simulink subsystem "HousegenTransform"  (R2023b)
settings: Solver=VariableStepAuto  StartTime=0.0  StopTime=10.0  RelTol=1e-3
libraries: hdlsllib x1
settings Model: Creator=Koche  LastModifiedBy=Koche

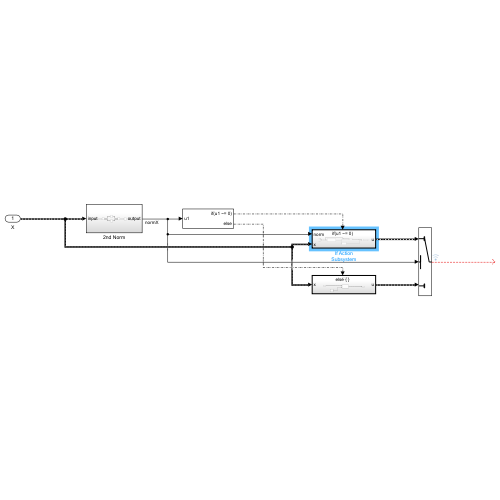
[thumbnail: Simulink's stored preview of the top-level diagram]
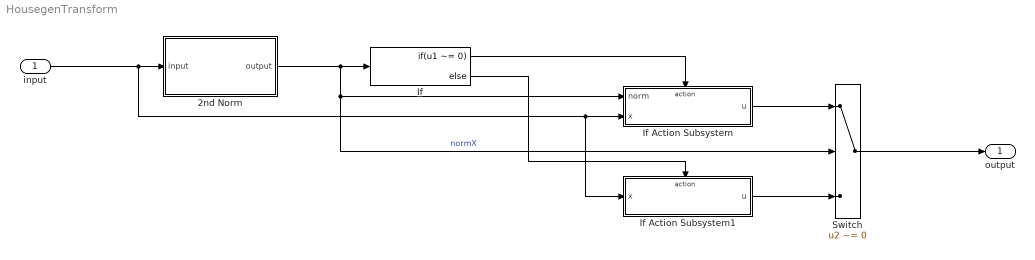
== system HousegenTransform ==
  input : Inport
  2nd Norm : Subsystem
  If : If  IfExpression=u1 ~= 0
  If Action Subsystem : Subsystem  TreatAsAtomicUnit=on
  If Action Subsystem1 : Subsystem  TreatAsAtomicUnit=on
  Switch : Switch  Criteria=u2 ~= 0  AllowDiffInputSizes=on  SaturateOnIntegerOverflow=off  InputSameDT=off
  output : Outport
  wires:
  Switch/1 -> output/1
  If/2 -> If Action Subsystem1/Action
  input/1 -> If Action Subsystem/2(x), If Action Subsystem1/1(x), 2nd Norm/1(input)
  2nd Norm/1(output) -> Switch/2, If Action Subsystem/1(norm), If/1  "normX"
  If Action Subsystem/1(u) -> Switch/1
  If/1 -> If Action Subsystem/Action
  If Action Subsystem1/1(u) -> Switch/3

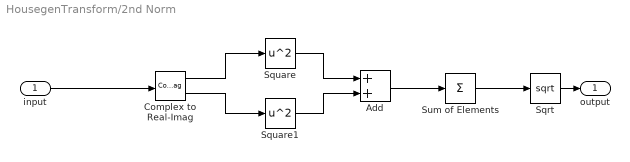
== system HousegenTransform/2nd Norm ==
  input : Inport
  Add : Sum
  Complex to Real-Imag : ComplexToRealImag
  Sqrt : Sqrt
  Square : Math  Operator=square  SignedPower=on  RndMeth=Zero
  Square1 : Math  Operator=square  SignedPower=on  RndMeth=Zero
  Sum of Elements : Sum  Inputs=+
  output : Outport
  wires:
  Square1/1 -> Add/2
  Sum of Elements/1 -> Sqrt/1
  Add/1 -> Sum of Elements/1
  Square/1 -> Add/1
  Complex to Real-Imag/1 -> Square/1
  Sqrt/1 -> output/1
  Complex to Real-Imag/2 -> Square1/1
  input/1 -> Complex to Real-Imag/1

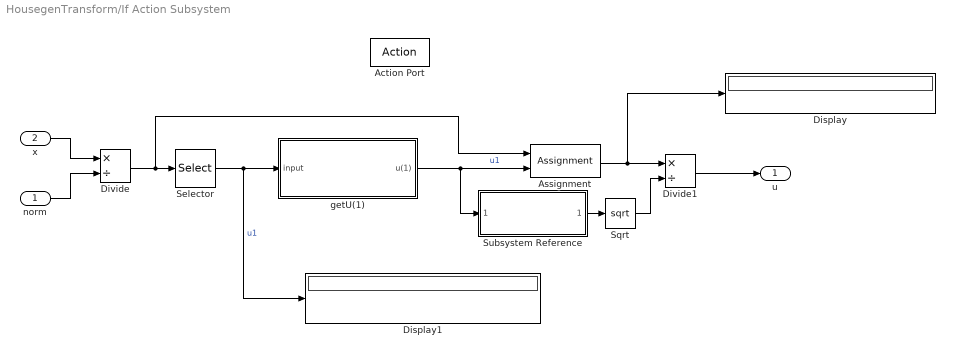
== system HousegenTransform/If Action Subsystem ==
  norm : Inport
  x : Inport  Port=2
  Action Port : ActionPort  InitializeStates=reset  PropagateVarSize=During execution
  Assignment : Assignment  IndexOptions=Index vector (dialog)  Indices=1  OutputSizes=1
  Display : Display
  Display1 : Display
  Divide : Product  Inputs=*/  RndMeth=Zero  SaturateOnIntegerOverflow=on
  Divide1 : Product  Inputs=*/  RndMeth=Zero  SaturateOnIntegerOverflow=on
  Selector : Selector  NumberOfDimensions=2  InputPortWidth=FrameLength  IndexOptions=Starting index (dialog),Index vector (dialog)  Indices=1,1  OutputSizes=1,1
  Sqrt : Sqrt
  Subsystem Reference : Subsystem  ReferencedSubsystem=CompAbs
  getU(1) : Subsystem
  u : Outport
  wires:
  Sqrt/1 -> Divide1/2
  Selector/1 -> getU(1)/1(input), Display1/1  "u1"
  x/1 -> Divide/1
  norm/1 -> Divide/2
  Divide/1 -> Selector/1, Assignment/1
  Divide1/1 -> u/1
  Subsystem Reference/1 -> Sqrt/1
  Assignment/1 -> Divide1/1, Display/1
  getU(1)/1(u(1)) -> Assignment/2, Subsystem Reference/1  "u1"

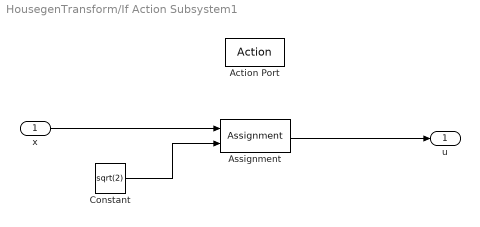
== system HousegenTransform/If Action Subsystem1 ==
  x : Inport
  Action Port : ActionPort  PropagateVarSize=During execution
  Assignment : Assignment  IndexOptions=Index vector (dialog)  Indices=1  OutputSizes=1
  Constant : Constant  Value=sqrt(2)
  u : Outport
  wires:
  x/1 -> Assignment/1
  Constant/1 -> Assignment/2
  Assignment/1 -> u/1

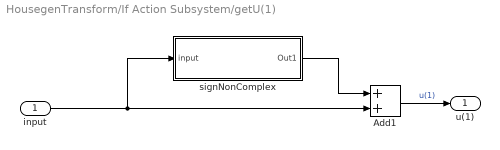
== system HousegenTransform/If Action Subsystem/getU(1) ==
  input : Inport
  Add1 : Sum
  signNonComplex : Subsystem
  u(1) : Outport
  wires:
  signNonComplex/1(Out1) -> Add1/1
  input/1 -> Add1/2, signNonComplex/1(input)
  Add1/1 -> u(1)/1  "u(1)"

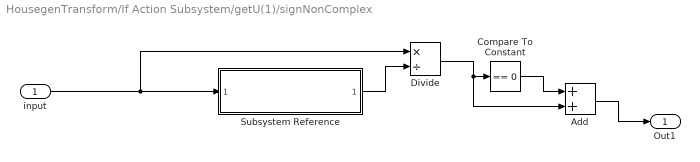
== system HousegenTransform/If Action Subsystem/getU(1)/signNonComplex ==
  input : Inport
  Add : Sum
  Compare To Constant : hdlsllib/Logic and Bit Operations/Compare To Constant  relop===  const=0  OutDataTypeStr=boolean
  Divide : Product  Inputs=*/  RndMeth=Zero  SaturateOnIntegerOverflow=on
  Subsystem Reference : Subsystem  ReferencedSubsystem=CompAbs
  Out1 : Outport
  wires:
  Subsystem Reference/1 -> Divide/2
  input/1 -> Subsystem Reference/1, Divide/1
  Add/1 -> Out1/1
  Compare To Constant/1 -> Add/1
  Divide/1 -> Add/2, Compare To Constant/1
